simulink model "ACDCAC"  (R2023b)
settings: Solver=VariableStepAuto  StartTime=0.0  StopTime=1  RelTol=1e-3
libraries: spsThreePhaseSeriesRLCBranchLib x4, simulink x3, spsThreePhaseVIMeasurementLib x2, spsUniversalBridgeLib x2, spsCurrentMeasurementLib x1, spsGroundLib x1, spsMultimeterLib x1, spsPWMGenerator2LevelLib x1, spsSeriesRLCBranchLib x1, spsThreePhaseSourceLib x1, sps_lib x1
settings Model: Creator=13615  LastModifiedBy=Tricycle Edson

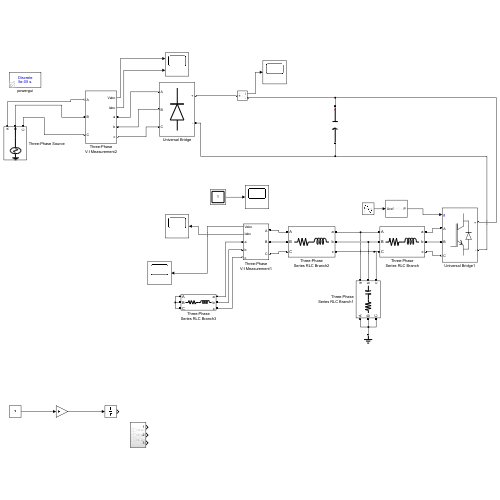
[thumbnail: Simulink's stored preview of the top-level diagram]
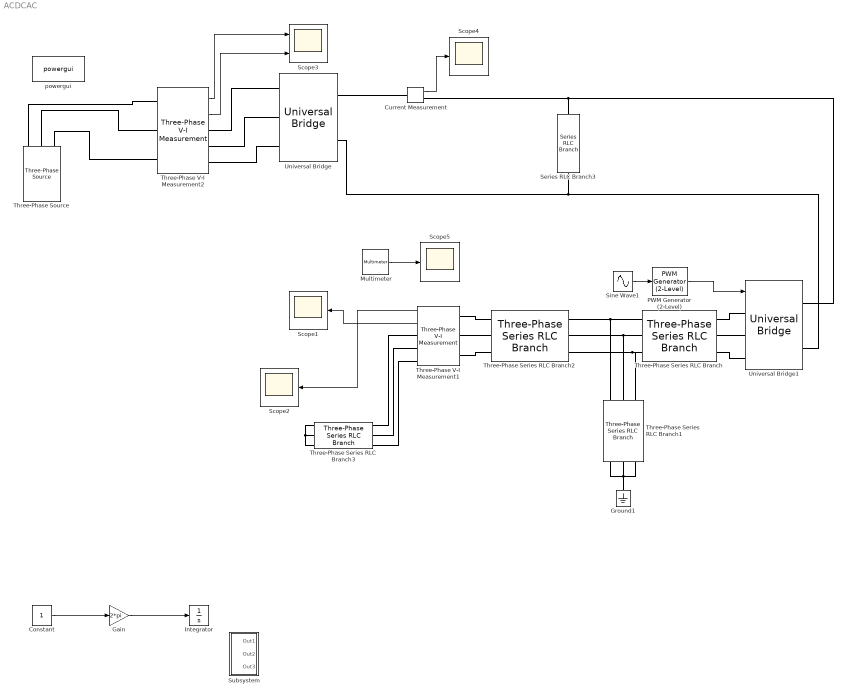
== system ACDCAC ==
  Constant : Constant
  Current Measurement : spsCurrentMeasurementLib/Current Measurement  PhasorSimulation=off  OutputType=Complex  PSBequivalent=0
  Gain : Gain  Gain=2*pi
  Ground1 : spsGroundLib/Ground  LConnTagsString=a
  Integrator : Integrator
  Multimeter : spsMultimeterLib/Multimeter  L=4  sel=4  yselected={}  Gain=1  OutputType=Complex  PlotAtSimulationStop=off  PhasorSimulation=off
  PWM Generator (2-Level) : spsPWMGenerator2LevelLib/PWM Generator (2-Level)  ModulatorType=Three-phase bridge (6 pulses)  ModulatorMode=Unsynchronized  Fc=90*50  Pc=90  nF=27  MinMax="[ -1  1 ]"  SamplingTechnique=Natural  ModulatingSignals=off  m=0.8  Freq=60  Phase=0  Ts=0  ShowCarrierOutport=off
  Scope{1..2,4..5} (4 alike) : Scope
  Scope3 : Scope  NumInputPorts=2
  Series RLC Branch3 : spsSeriesRLCBranchLib/Series RLC Branch  LConnTagsString=__new0  RConnTagsString=__new0  BranchType=C  Resistance=0  Inductance=0  SetiL0=off  InitialCurrent=0  Capacitance=50e-5  Setx0=off  InitialVoltage=0  Measurements=None
  Sine Wave1 : Sin  Frequency=50*2*pi  Phase=[0 (2/3)*pi -(2/3)*pi]  SampleTime=0
  Subsystem : Subsystem
  Three-Phase Series RLC Branch : spsThreePhaseSeriesRLCBranchLib/Three-Phase Series RLC Branch  LConnTagsString=A|B|C  RConnTagsString=A|B|C  BranchType=RL  Resistance=0.01  Inductance=300e-4  Capacitance=1e-6  Measurements=None
  Three-Phase Series RLC Branch1 : spsThreePhaseSeriesRLCBranchLib/Three-Phase Series RLC Branch  LConnTagsString=A|B|C  RConnTagsString=A|B|C  BranchType=RC  Resistance=0.01  Inductance=1e-3  Capacitance=500e-6  Measurements=None
  Three-Phase Series RLC Branch2 : spsThreePhaseSeriesRLCBranchLib/Three-Phase Series RLC Branch  LConnTagsString=A|B|C  RConnTagsString=A|B|C  BranchType=RL  Resistance=0.01  Inductance=300e-4  Capacitance=1e-6  Measurements=None
  Three-Phase Series RLC Branch3 : spsThreePhaseSeriesRLCBranchLib/Three-Phase Series RLC Branch  LConnTagsString=A|B|C  RConnTagsString=A|B|C  BranchType=RL  Resistance=20  Inductance=500e-5  Capacitance=1e-6  Measurements=None
  Three-Phase V-I Measurement1 : spsThreePhaseVIMeasurementLib/Three-Phase V-I Measurement  VoltageMeasurement=phase-to-ground  SetLabelV=off  LabelV=Vabc  Vpu=off  VpuLL=off  CurrentMeasurement=yes  SetLabelI=off  LabelI=Iabc  Ipu=off  Pbase=100e6  Vbase=500e3  OutputType=Complex  PhasorSimulation=off  PSBequivalent=0
  Three-Phase V-I Measurement2 : spsThreePhaseVIMeasurementLib/Three-Phase V-I Measurement  VoltageMeasurement=phase-to-ground  SetLabelV=off  LabelV=Vabc  Vpu=off  VpuLL=off  CurrentMeasurement=yes  SetLabelI=off  LabelI=Iabc  Ipu=off  Pbase=100e6  Vbase=500e3  OutputType=Complex  PhasorSimulation=off  PSBequivalent=0
  Three-Phase Source : spsThreePhaseSourceLib/Three-Phase Source  InternalConnection=Yg  VoltagePhases=off  Voltage=380  PhaseAngle=0  Voltage_phases=[25e3 25e3 25e3]/sqrt(3)  PhaseAngles_phases=[0 -120 +120]  Frequency=50  NonIdealSource=on  SpecifyImpedance=off  Resistance=0  Inductance=0  ShortCircuitLevel=100e6  BaseVoltage=380  XRratio=7  BusType=swing  Pref=10e3  Qref=0  Prefabc=[10e3, 10e3, 10e3]  Qrefabc=[0, 0, 0]  Qmin=-inf  Qmax=inf
  Universal Bridge : spsUniversalBridgeLib/Universal Bridge  Arms=3  SnubberResistance=1e5  SnubberCapacitance=inf  Device=Diodes  Ron=1e-3  Lon=0  ForwardVoltages="[  0  0  ]"  ForwardVoltage=0  GTOparameters=[ 10e-6 , 20e-6 ]  IGBTparameters=[ 1e-6 , 2e-6 ]  Measurements=UAB UBC UCA UDC voltages  Measurements_2=None  converterType=Rectifier
  Universal Bridge1 : spsUniversalBridgeLib/Universal Bridge  Arms=3  SnubberResistance=1e5  SnubberCapacitance=inf  Device=IGBT / Diodes  Ron=1e-3  Lon=0  ForwardVoltages="[  0  0  ]"  ForwardVoltage=0  GTOparameters=[ 10e-6 , 20e-6 ]  IGBTparameters=[ 1e-6 , 2e-6 ]  Measurements=None  Measurements_2=None  converterType=Rectifier
  powergui : sps_lib/powergui  Priority=1  SimulationMode=Discrete  SampleTime=50e-6  frequency=60  Iterations=50  frequencyindice=50  Pbase=100e6  ErrMax=1e-4  UnitsV=kV  UnitsW=MW  buscounter=0  FunctionMessages=off  echomessages=off  EnableUseOfTLC=off  CurrentSourceSwitches=off  DisableSnubberDevices=off  DisableRonSwitches=off  DisableVfSwitches=off  DisplayEquations=off  AutomaticDiscreteSolvers=off  SolverType=Tustin/Backward Euler (TBE)  Interpol=off  ExternalGateDelay=off  methode=off  Ts=100  x0status=blocks  SPID=on  SwTol=0  HookPort=off  NonlinearTolerance=1e-4  nMaxIteration=100  ContinueOnMaxIteration=off  RestoreLinks=warning  ResistiveCurrentMeasurement=off  Frange=[0:2:500]  Ylog=off  Xlog=on  ShowGrid=off  save=off  variable=ZData  structure=0  ZoomFFT=off  StartTime=0.0  cycles=1  DisplayStyle=1  fundamental=60  FreqAxis=off  MaxFrequency=1000  frequencyindicesteady=1  RmsSteady=1  display=off
  wires:
  Constant/1 -> Gain/1
  Gain/1 -> Integrator/1
  Sine Wave1/1 -> PWM Generator (2-Level)/1
  PWM Generator (2-Level)/1 -> Universal Bridge1/1
  Three-Phase V-I Measurement1/2 -> Scope1/1
  Three-Phase V-I Measurement1/1 -> Scope2/1
  Three-Phase V-I Measurement2/2 -> Scope3/2
  Three-Phase V-I Measurement2/1 -> Scope3/1
  Current Measurement/1 -> Scope4/1
  Multimeter/1 -> Scope5/1
  connections:
  Universal Bridge1/LConn1 -- Three-Phase Series RLC Branch/RConn1
  Universal Bridge1/LConn2 -- Three-Phase Series RLC Branch/RConn2
  Universal Bridge1/LConn3 -- Three-Phase Series RLC Branch/RConn3
  Three-Phase Series RLC Branch1/RConn1 -- Three-Phase Series RLC Branch/LConn1 -- Three-Phase Series RLC Branch2/RConn1
  Three-Phase Series RLC Branch1/RConn2 -- Three-Phase Series RLC Branch2/RConn2 -- Three-Phase Series RLC Branch/LConn2
  Three-Phase Series RLC Branch/LConn3 -- Three-Phase Series RLC Branch2/RConn3 -- Three-Phase Series RLC Branch1/RConn3
  Three-Phase V-I Measurement1/LConn1 -- Three-Phase Series RLC Branch2/LConn1
  Three-Phase Series RLC Branch2/LConn2 -- Three-Phase V-I Measurement1/LConn2
  Three-Phase V-I Measurement1/LConn3 -- Three-Phase Series RLC Branch2/LConn3
  Universal Bridge/RConn1 -- Current Measurement/LConn1
  Universal Bridge1/RConn2 -- Series RLC Branch3/RConn1 -- Universal Bridge/RConn2
  Series RLC Branch3/LConn1 -- Universal Bridge1/RConn1 -- Current Measurement/RConn1
  Three-Phase Series RLC Branch1/LConn1 -- Ground1/LConn1 -- Three-Phase Series RLC Branch1/LConn2 -- Three-Phase Series RLC Branch1/LConn3
  Three-Phase Series RLC Branch3/RConn2 -- Three-Phase V-I Measurement1/RConn2
  Three-Phase V-I Measurement1/RConn1 -- Three-Phase Series RLC Branch3/RConn1
  Three-Phase V-I Measurement1/RConn3 -- Three-Phase Series RLC Branch3/RConn3
  Three-Phase Series RLC Branch3/LConn1 -- Three-Phase Series RLC Branch3/LConn3 -- Three-Phase Series RLC Branch3/LConn2
  Three-Phase V-I Measurement2/RConn3 -- Universal Bridge/LConn3
  Three-Phase V-I Measurement2/RConn2 -- Universal Bridge/LConn2
  Three-Phase V-I Measurement2/RConn1 -- Universal Bridge/LConn1
  Three-Phase Source/RConn1 -- Three-Phase V-I Measurement2/LConn1
  Three-Phase Source/RConn2 -- Three-Phase V-I Measurement2/LConn2
  Three-Phase Source/RConn3 -- Three-Phase V-I Measurement2/LConn3

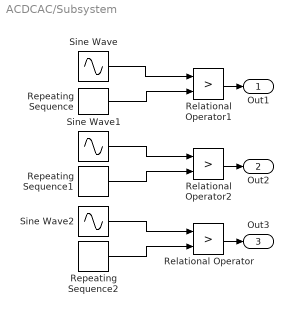
== system ACDCAC/Subsystem ==
  Relational Operator : RelationalOperator  Operator=>  OutDataTypeStr=boolean  RndMeth=Simplest  InputSameDT=off
  Relational Operator1 : RelationalOperator  Operator=>  OutDataTypeStr=boolean  RndMeth=Simplest  InputSameDT=off
  Relational Operator2 : RelationalOperator  Operator=>  OutDataTypeStr=boolean  RndMeth=Simplest  InputSameDT=off
  Repeating Sequence : simulink/Sources/Repeating Sequence  rep_seq_t=[0 1 2]  rep_seq_y=[1 -1 1]
  Repeating Sequence1 : simulink/Sources/Repeating Sequence  rep_seq_t=[0 1 2]  rep_seq_y=[1 -1 1]
  Repeating Sequence2 : simulink/Sources/Repeating Sequence  rep_seq_t=[0 1 2]  rep_seq_y=[1 -1 1]
  Sine Wave : Sin  SampleTime=0
  Sine Wave1 : Sin  Phase=2/3*pi  SampleTime=0
  Sine Wave2 : Sin  Phase=-2/3*pi  SampleTime=0
  Out1 : Outport
  Out2 : Outport  Port=2
  Out3 : Outport  Port=3
  wires:
  Relational Operator/1 -> Out3/1
  Sine Wave/1 -> Relational Operator1/1
  Repeating Sequence2/1 -> Relational Operator/2
  Relational Operator1/1 -> Out1/1
  Sine Wave2/1 -> Relational Operator/1
  Repeating Sequence1/1 -> Relational Operator2/2
  Repeating Sequence/1 -> Relational Operator1/2
  Sine Wave1/1 -> Relational Operator2/1
  Relational Operator2/1 -> Out2/1
